simulink model "gripper_model"  (R2021a)
settings: Solver=ode15s  StartTime=0.0  StopTime=3  FixedStep=0.0001  RelTol=0.01
InitFcn:
  | p_init;
values from neighbouring files (symbols this model uses):
  a_w = 0    [p_init_wrist.m]
  B_r_w = t_0_w/w_0_w    (= 1.76664947854e-08)    [p_init_wrist.m]
  b_w = 1/1.34e6    (= 7.46268656716e-07)    [p_init_wrist.m]
  J_a_w = 0.0000515    (= 5.15e-05)    [p_init_wrist.m]
  J_r_w = 0.035 * 1e-7    (= 3.5e-09)    [p_init_wrist.m]
  K_b_w = 1/(1100*2*pi/60)    (= 0.0086811787141)    [p_init_wrist.m]
  K_m_w = 8.71 / 1000    (= 0.00871)    [p_init_wrist.m]
  K_p_w = 4.72e6/1.34e6    (= 3.5223880597)    [p_init_wrist.m]
  L_term_w = 0.276 / 1000    (= 0.000276)    [p_init_wrist.m]
  R_term_w = 92.2    [p_init_wrist.m]
  v_max_amp_w = +V_nom_w    (= 12)    [p_init_wrist.m]
  v_min_amp_w = -V_nom_w    (= -12)    [p_init_wrist.m]
libraries: pid_lib x1
settings Model: Creator=Konstantin  LastModifiedBy=kossio
settings SolverCC: ZeroCrossControl=DisableAll  AlgebraicLoopSolver=TrustRegion
settings DebuggingCC: SFMachineParentedDataDiag=warning

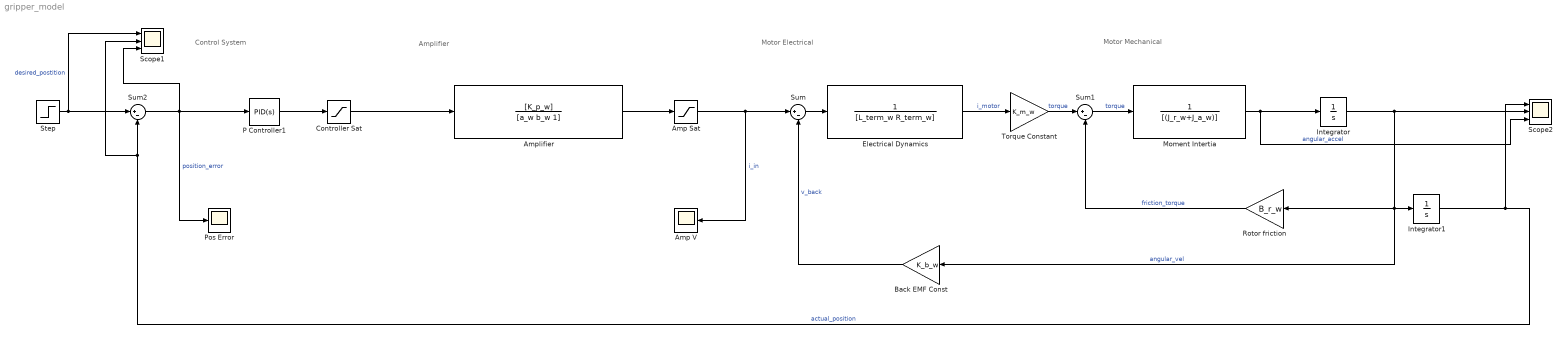
== system gripper_model ==
  note: Control System
  note: Motor Mechanical
  note: Motor Electrical
  note: Amplifier
  Amp Sat : Saturate  UpperLimit=v_max_amp_w  LowerLimit=v_min_amp_w
  Amp V : Scope
  Amplifier : TransferFcn  Numerator=[K_p_w]  Denominator=[a_w b_w 1]
  Back EMF Const : Gain  Gain=K_b_w
  Controller Sat : Saturate  UpperLimit=10  LowerLimit=-10
  Electrical Dynamics : TransferFcn  Denominator=[L_term_w R_term_w]
  Integrator : Integrator
  Integrator1 : Integrator
  Moment Intertia : TransferFcn  Denominator=[(J_r_w+J_a_w)]
  P Controller1 : pid_lib/PID Controller  Controller=PID  Form=Parallel  TimeDomain=Continuous-time  UseExternalTs=off  SampleTime=-1  IntegratorMethod=Forward Euler  FilterMethod=Forward Euler  ControllerParametersSource=internal  P=1  I=0  D=0  UseFilter=on  N=100  TunerSelectOption=Transfer Function Based (PID Tuner App)  InitialConditionSource=internal  InitialConditionForIntegrator=0  InitialConditionForFilter=0  DifferentiatorICPrevScaledInput=0  ExternalReset=none  TrackingMode=off  Kt=1  LimitOutput=off  SatLimitsSource=internal  UpperSaturationLimit=inf  LowerSaturationLimit=-inf  LinearizeAsGain=on  AntiWindupMode=none  Kb=1  POutMin=[]  POutMax=[]  IOutMin=[]  IOutMax=[]  DOutMin=[]  DOutMax=[]  NOutMin=[]  NOutMax=[]  SumOutMin=[]  SumOutMax=[]  SaturationOutMin=[]  SaturationOutMax=[]  PParamMin=[]  PParamMax=[]  IParamMin=[]  IParamMax=[]  DParamMin=[]  DParamMax=[]  NParamMin=[]  NParamMax=[]  KbParamMin=[]  KbParamMax=[]  KtParamMin=[]  KtParamMax=[]  KbOutMin=[]  KbOutMax=[]  KtOutMin=[]  KtOutMax=[]  IntegratorOutMin=[]  IntegratorOutMax=[]  FilterOutMin=[]  FilterOutMax=[]  SumI1OutMin=[]  SumI1OutMax=[]  SumI2OutMin=[]  SumI2OutMax=[]  SumI3OutMin=[]  SumI3OutMax=[]  SumI4OutMin=[]  SumI4OutMax=[]  SumDOutMin=[]  SumDOutMax=[]  DifferentiatorOutMin=[]  DifferentiatorOutMax=[]  FilterDiffOutCoefMin=[]  FilterDiffOutCoefMax=[]  ReciprocalOutMin=[]  ReciprocalOutMax=[]  SumDenOutMin=[]  SumDenOutMax=[]  SumNumOutMin=[]  SumNumOutMax=[]  DivideOutMin=[]  DivideOutMax=[]  UdiffTsProdOutMin=[]  UdiffTsProdOutMax=[]  NTsProdOutMin=[]  NTsProdOutMax=[]  UintegralTsProdOutMin=[]  UintegralTsProdOutMax=[]  UngainTsProdOutMin=[]  UngainTsProdOutMax=[]  IntegratorContinuousStateAttributes=''  IntegratorStateMustResolveToSignalObject=off  IntegratorRTWStateStorageClass=Auto  FilterContinuousStateAttributes=''  FilterStateMustResolveToSignalObject=off  FilterRTWStateStorageClass=Auto  ParallelPVariant=InternalParameters  IdealPVariant=Disabled  IVariant=InternalParameters  DVariant=InternalParameters  IntegratorVariant=Continuous  SatVariant=Disabled  AWVariant=Passthrough  PCopyVariant=Disabled  TRVariant=Disabled  FdbkBlocksVariant=Forward  IdealPFdbkVariant=Disabled  SatFdbkVariant=Disabled  DerivativeFilterVariant=ContFilter  NVariant=InternalParameters  NCopyVariant=Disabled  FilterICVariant=InternalICsFilter  IntegratorICVariant=InternalICs  ExternalResetVariant=Disabled  TRSumVariant=Passthrough  SumFdbkVariant=Disabled  SumVariant=Sum_PID  TsampFilterVariant=InternalTs  TsampNgainVariant=Passthrough  TsampIntegralVariant=Passthrough  ExternalSaturationOutDataTypeStr=Inherit: Same as second input
  Pos Error : Scope
  Rotor friction : Gain  Gain=B_r_w
  Scope1 : Scope  NumInputPorts=3
  Scope2 : Scope  NumInputPorts=3
  Step : Step  Time=0  After=pi/2  SampleTime=0
  Sum : Sum  Inputs=|+-
  Sum1 : Sum  Inputs=|+-
  Sum2 : Sum  Inputs=|+-
  Torque Constant : Gain  Gain=K_m_w
  wires:
  Sum/1 -> Electrical Dynamics/1
  Electrical Dynamics/1 -> Torque Constant/1  "i_motor"
  Amp Sat/1 -> Amp V/1, Sum/1  "i_in"
  Back EMF Const/1 -> Sum/2  "v_back"
  Moment Intertia/1 -> Scope2/3, Integrator/1  "angular_accel"
  Integrator/1 -> Scope2/2, Back EMF Const/1, Integrator1/1, Rotor friction/1  "angular_vel"
  Rotor friction/1 -> Sum1/2  "friction_torque"
  Torque Constant/1 -> Sum1/1  "torque"
  Sum1/1 -> Moment Intertia/1  "torque"
  Step/1 -> Sum2/1, Scope1/1  "desired_postition"
  Integrator1/1 -> Sum2/2, Scope1/2, Scope2/1  "actual_position"
  Controller Sat/1 -> Amplifier/1
  Amplifier/1 -> Amp Sat/1
  Sum2/1 -> P Controller1/1, Scope1/3, Pos Error/1  "position_error"
  P Controller1/1 -> Controller Sat/1
